simulink model "WaveBot3Dof_Control"  (R2022b)
settings: Solver=ode45  StartTime=0  StopTime=1200  FixedStep=0.01  MaxStep=0.01  RelTol=1e-3
values from neighbouring files (symbols this model uses):
  adaptSlope = [1e-4, 1e-4, 1e-3; 5e-7, 5e-7, 5e-4]    [wecSimInputFile.m]
  FBEnable = 1    [wecSimInputFile.m]
  FFEnable = 0    [wecSimInputFile.m]
  gear_ratio_h = 12.4666    [wecSimInputFile.m]
  gear_ratio_sp = diag([12.4666, 3])    [wecSimInputFile.m]
  intGain = [0, 5e-7, 1e-7; 0 5e-6 5e-8; 0 5e-5 5e-7]    [wecSimInputFile.m]
  K = 10.96    [wecSimInputFile.m]
  Kt_h = 6.1745    [wecSimInputFile.m]
  Kt_sp = 6.1745 * eye(2)    [wecSimInputFile.m]
  m = 3    [wecSimInputFile.m]
  N_max = floor(spect.f_max/spect.df)    [wecSimInputFile.m]
  N_min = ceil(spect.f_min/spect.df)    [wecSimInputFile.m]
  objCase = 1    [wecSimInputFile.m]
  OpenLoopGains = [50;100;2]    [wecSimInputFile.m]
  R_h = 0.5    [wecSimInputFile.m]
  R_sp = diag([0.5,  0.5])    [wecSimInputFile.m]
  simu = simulationClass()    [wecSimInputFile.m]
  T = 300    [wecSimInputFile.m]
  threshDF = [6000;8000;375]    [wecSimInputFile.m]
  threshPTO = [1200;1200;150]    [wecSimInputFile.m]
  Ts = dt    (= 0.01)    [wecSimInputFile.m]
  w = 2*pi*spect.f.'    [wecSimInputFile.m]
  WeightAdapt = 0    [wecSimInputFile.m]
  WeightCase = [25, 0.2,0.01; 25,0.1,0.01;25,0.2,0.1]    [wecSimInputFile.m]
  Z = [931.288383881 1656.98600833 760.743138043 168.271740533 368.778972104 366.885270862 -556.942327031 -1377.9298451 -1305.0085586 758.156793041 1688.7138346 185.859065593 ... (4023 elements, 3x3x447)]    [Z_included.mat]
  Zi_frf_AT = interp_impedance(Z,f_vec*2*pi,w)    [wecSimInputFile.m]
undefined symbols (not defined in the file or in its folder): body, constraint, Constraints, DiscIntNeverNeededParam, Floating, geometry, hydroData, mooring, spect, WECSim_Lib, WECSim_Lib_Constraints, X, Y
libraries: nesl_utility x28, sm_lib x14, simulink x6, WECSim_Lib_Frames x1, WECSim_Lib_Moorings x1, WECSim_Lib_Body_Elements x1, dspxfrm3 x1, matrix_library x1, dspsigops x1
(part 2 of 2)

== system WaveBot3Dof_Control/Subsystem/Autotuner/PTO Weight Integrator Logic/Triggered Subsystem ==
  Trigger : TriggerPort  VariantControl=Variant
  Constant : Constant  Value=0
  Constant1 : Constant
  Plus : Sum
  Out1 : Outport
  wires:
  Plus/1 -> Out1/1
  Constant/1 -> Plus/2
  Constant1/1 -> Plus/1

== system WaveBot3Dof_Control/Subsystem/Autotuner/PTO Weight Integrator Logic/Triggered Subsystem1 ==
  Trigger : TriggerPort  VariantControl=Variant
  Constant : Constant  Value=0
  Constant1 : Constant
  Plus : Sum
  Out1 : Outport
  wires:
  Plus/1 -> Out1/1
  Constant/1 -> Plus/2
  Constant1/1 -> Plus/1

== system WaveBot3Dof_Control/Subsystem/Autotuner/PTO Weight Integrator Logic/Triggered Subsystem2 ==
  Trigger : TriggerPort  VariantControl=Variant
  Constant : Constant  Value=0
  Constant1 : Constant
  Plus : Sum
  Out1 : Outport
  wires:
  Plus/1 -> Out1/1
  Constant/1 -> Plus/2
  Constant1/1 -> Plus/1

== matlab function WaveBot3Dof_Control/Subsystem/Subsystem/MATLAB Function ==
  data: vel input; Fdes output; pos input; gains input
function Fdes = PI_D_Controller(vel,pos,gains)

Fdes = zeros(3,1); % initialize output
Kp = zeros(3,1);
Ki = zeros(3,1);
D = zeros(3,1);
K = zeros(3,1); 

% build control vectors
Kp(:,1) = gains(1:2:5);
Ki(:,1) = gains(2:2:6);

% multiply elementwise by vel, pos
D = Kp .* vel;
K = Ki .* pos;

% sum according to convention
Fdes = D + K;

== matlab function WaveBot3Dof_Control/Subsystem/Autotuner/Spectral Estimation/MATLAB Function ==
  data: in1 input; Fexc output; Zi_frf_AT parameter
function Fexc = fcn(in1,  Zi_frf_AT)

F = in1(:,4:6);
V = in1(:,1:3);

Fexc = 0*F(:,[1:3]);%zeros(1,spect.N_freq);

for ii = 1:length(Fexc)
    
    % use heave only estimate 
    %Fexc(ii,1) = 2 *( Y_inv(1,:,ii)*V(ii,:).' - F(ii,1).' );%* H_inv(ii,:)
    
    % use full estimate
    Fexc(ii,:) = 2 *( Zi_frf_AT(:,:,ii)*V(ii,:).' - F(ii,:).' );
    % ETA(ii) = [1,1,1]*Y_inv(:,:,ii)*V(ii,:).';
end

% ETA = F;

== matlab function WaveBot3Dof_Control/Subsystem/Autotuner/MATLAB Function1 ==
  data: Fe input; optGains output; initGuess input; nextInit output; Kt_h parameter; R_h parameter; w parameter; Zi_frf_AT parameter; gear_ratio_h parameter; Kt_sp parameter; R_sp parameter; gear_ratio_sp parameter; m parameter; K parameter; T parameter; Weights input; PTO_h output; PTO_sp output; Df_h output; Df_sp output
function [optGains,nextInit, PTO_h, PTO_sp, Df_h, Df_sp] = gainOptimizer(Fe,initGuess,...
    Kt_h,R_h, w, Zi_frf_AT, gear_ratio_h, Kt_sp, R_sp, gear_ratio_sp, m, K, T, Weights)
% R_h = 0;
% unfortunately we must declare options every time we run
options = optimset('Display','off', 'MaxFunEvals', 1e4, 'MaxIter', 1e4);%
% further, apparently code generation cannot handle specified TolX and
% TolFun. Defaults, however, do seem adequate.

% initialize:
optGains=zeros(6,1); % initialize estimate (6 for diag only, 8 for CC)
nextInit=optGains;
cost_h = 1i; cost_sp = 1i;
exitFlag_h = 0; exitFlag_sp = 0; 
PTO_h = 0 ;
PT0_sp = zeros(2,1);
Df_h = 0; 
Df_sp = zeros(2,1);

%% break up impedance model by DOF '

% for heave only (this is not coupled to other DOFs)
Zi_frf_h=Zi_frf_AT(2,2,:);

% for surge and pitch (these are coupled)
Zi_frf_sp=Zi_frf_AT([1,3],[1,3],:);

% transpose necessary for dimensions to work out
Fe_h=Fe(:,2).';
Fe_sp=Fe(:,[1,3]).';

%% set up optimizer
cost_fun_h = @(x_h) WaveBot_power(Zi_frf_h, Fe_h, ...
    PI_FB_SISO_controller_FRF(x_h, w) , Kt_h, R_h, gear_ratio_h,Weights, m, K, T,w);

% optimize heave controller
[optGains([3,4],1)]= fminsearch(cost_fun_h, [-1000,500], options); % here a static initial guess is used: during sim ramp-up changing initial guess can be unstable

cost_fun_sp_d=@(x_sp) WaveBot_power(Zi_frf_sp, Fe_sp,...
    PI_FB_MIMO_D_controller_FRF(x_sp, w) , Kt_sp, R_sp, gear_ratio_sp,Weights, m, K, T,[w,w]);

% optimize surge/pitch controller
[optGains([1,2,5,6],1)]=fminsearch(cost_fun_sp_d, initGuess([1,2,5,6],1), options);

% output spectral info for weight adjustment
[~, ~, ~, ~, PTO_h, Df_h] = WaveBot_powerH(Zi_frf_h,Fe_h,PI_FB_SISO_controller_FRF(optGains([3,4],1), w), Kt_h, R_h, gear_ratio_h, Weights, m, K, T, w);
[~, ~, ~, ~, PTO_sp, Df_sp] = WaveBot_powerSP(Zi_frf_sp,Fe_sp, PI_FB_MIMO_D_controller_FRF(optGains([1,2,5,6],1), w), Kt_sp, R_sp, gear_ratio_sp, Weights, m, K, T, [w,w]);

% update initial guess for next time
nextInit=optGains;

% Single input single output controller for heave
    function C_h = PI_FB_SISO_controller_FRF(x_h, w)
        C_h=1i*ones(1,1,length(w)); 
        
        Kp = x_h(1);
        Ki = x_h(2);
        w = w(:);
        
        C_h(1,1,:) = Kp - 1i*Ki./w;
        
    end

% 2 input 2 output controller for surge-pitch control
    function C_sp = PI_FB_MIMO_D_controller_FRF(x_sp, w)
        C_sp=1i*ones(2,2,length(w)); C_sp(2,1)=0; C_sp(1,2)=C_sp(2,1);
        
        Kp_s = x_sp(1);
        Ki_s = x_sp(2);
        Kp_p = x_sp(3);
        Ki_p = x_sp(4);
        w = w(:);

        C_sp(1,1,:) = Kp_s - 1i*Ki_s./w;
        C_sp(2,2,:) = Kp_p - 1i*Ki_p./w;
    end
 
% optimizer runs this version
 function [Cost2, P, Cost1, Omega, Loads, Df]= WaveBot_power(Zi, Fe, C, Kt, R, gear_ratio, Weights, m, K, T, w)
        
     % initialize
        N_freq = size(Zi,3);
        P=0;
        P_f = 1i*ones(N_freq,1);
        Omega = 1i*ones(length(R),N_freq);
        Df = 0; 
        CF = 1i * ones(length(R),N_freq);
        TF = 1i * ones(length(R),N_freq);
        m0=0; 
        m2= 0; 
        v_up = 0; 
        Loads = 0; 
        Cost1 = 0; 
        Cost2 = 0; 
        
        if length(R)>1
            Weights2=Weights([1,3],:);  % if 2 DOF, pulls surge/pitch weights 
            Weights2(2,end) = -1.* Weights2(2,end);
        else
            Weights2=Weights(2,:);% if 1 DOF, pulls heave weights
        end
            Ke = Kt*2/3;
        
        for ii = 1:N_freq
            
            Omega(:,ii) = ( Zi(:,:,ii) - C(:,:,ii)) \ Fe(:,ii);
            P_f(ii) = ( (Ke*gear_ratio + (R/(gear_ratio*Kt))*C(:,:,ii)) * Omega(:,ii) )'...
                * ( ((gear_ratio*Kt)\C(:,:,ii)*Omega(:,ii)) );
            CF(:,ii)=abs(C(:,:,ii)*Omega(:,ii)); % controller force
            TF(:,ii)=(Fe(:,ii) + C(:,:,ii)*Omega(:,ii)); % total force
        end
        
        % calculate spectral moments of stress spectra
        m0 = trapz(w(:,1),abs(TF).^2,2);
        m2 = trapz(w(:,1),w.^2 .* abs((TF).^2).').';
        
        %calculate mean upcrossing time
        v_up = (1./(2*pi)).*sqrt(m2./m0);
        
        % calculate the standard deviation of the process
        sigma = sqrt(m0./length(w));
        
        % calculate the accumulated fatigue damage
        Df = (v_up.*T./K) .* (2*sqrt(2) .* sigma).^m .* gamma((m/2)+1);
        
        % calculate cost function
        P = sum(real(P_f))*3;
        Loads = sum(CF,2);
        Cost1 = real(Weights2(1,1)*P + Weights2(:,2).'*Loads);
        Cost2 = real(Weights2(1,1)*P + Weights2(:,2).'*Loads + Weights2(:,3).'*Df); 

 end

% the next two functions are basically repeats of the above, but are
% necessary to avoid size errors by the simulink code compiler

function [Cost2, P, Cost1, Omega, Loads, Df]= WaveBot_powerH(Zi, Fe, C, Kt, R, gear_ratio, Weights, m, K, T, w)
        % this includes all equally weighted loads
        % N_dof = length(R);
        % initialize all parameters/outputs
        N_freq = size(Zi,3);
        P=0;
        P_f = 1i*ones(N_freq,1);
        Omega = 1i*ones(length(R),N_freq);
        Df = 0; 
        CF = 1i * ones(length(R),N_freq);
        TF = 1i * ones(length(R),N_freq);
        sigma = 0;
        m0 = 0; 
        m2 = 0; 
        v_up = 0; 
        Loads = 0;
        Cost1 = 0; 
        Cost2 = 0;
        
        if length(R)>1
            Weights2=Weights([1,3],:); % if 2 DOF, pulls surge/pitch weights 
            Weights2(2,end) = -1.* Weights2(2,end); % to align with WS sign convention on pitch force
        else
            Weights2=Weights(2,:); % if 1 DOF, pulls heave weights
        end
            Ke = Kt*2/3;
        
        for ii = 1:N_freq
            
            Omega(:,ii) = ( Zi(:,:,ii) - C(:,:,ii)) \ Fe(:,ii);
            P_f(ii) = ( (Ke*gear_ratio + (R/(gear_ratio*Kt))*C(:,:,ii)) * Omega(:,ii) )'...
                * ( ((gear_ratio*Kt)\C(:,:,ii)*Omega(:,ii)) );
            CF(:,ii)=abs(C(:,:,ii)*Omega(:,ii)); % controller force
            TF(:,ii)=(Fe(:,ii) + C(:,:,ii)*Omega(:,ii)); % total force
        end
        
        % calculate spectral moments of stress spectra
        m0 = trapz(w(:,1),abs(TF).^2,2);
        m2 = trapz(w(:,1),w.^2 .* abs((TF).^2).').';
        
        %calculate mean upcrossing time
        v_up = (1./(2*pi)).*sqrt(m2./m0);
        
        % calculate the standard deviation of the process
        sigma = sqrt(m0./length(w));
        
        % calculate the accumulated fatigue damage
        Df = (v_up.*T./K) .* (2*sqrt(2) .* sigma).^m .* gamma((m/2)+1);
        
        if isnan(Df); % this catches the zero excitation case, which has an undefined zero-crossing time v_up
            Df = 0;
        end
        
        P = double(sum(real(P_f))*3);
        Loads = real(sum(CF,2));
        Cost1 = real(Weights2(1,1)*P + Weights2(:,2).'*Loads);
        Cost2 = real(Weights2(1,1)*P + Weights2(:,2).'*Loads + Weights2(:,3).'*Df); % additional penalty for reactive terms.
    end

function [Cost2, P, Cost1, Omega, Loads, Df]= WaveBot_powerSP(Zi, Fe, C, Kt, R, gear_ratio, Weights, m, K, T, w)

        N_freq = size(Zi,3);
        P=0;
        P_f = 1i*ones(N_freq,1);
        Omega = 1i*ones(length(R),N_freq);
        Df = zeros(2,1); 
        CF = 1i * ones(length(R),N_freq);
        TF = 1i * ones(length(R),N_freq);
        sigma = zeros(2,1);
        m0 = zeros(2,1); 
        m2 = zeros(2,1); 
        v_up = zeros(2,1); 
        Loads = zeros(2,1);
        Cost1 = zeros(2,1); 
        Cost2 = zeros(2,1);
        
        if length(R)>1
            Weights2=Weights([1,3],:);
            Weights2(2,end) = -1.* Weights2(2,end);
        else
            Weights2=Weights(2,:);
        end
            Ke = Kt*2/3;
        
        for ii = 1:N_freq
            
            Omega(:,ii) = ( Zi(:,:,ii) - C(:,:,ii)) \ Fe(:,ii);
            P_f(ii) = ( (Ke*gear_ratio + (R/(gear_ratio*Kt))*C(:,:,ii)) * Omega(:,ii) )'...
                * ( ((gear_ratio*Kt)\C(:,:,ii)*Omega(:,ii)) );
            CF(:,ii)=abs(C(:,:,ii)*Omega(:,ii)); % controller force
            TF(:,ii)=(Fe(:,ii) + C(:,:,ii)*Omega(:,ii)); % total force
        end
        
        % calculate spectral moments of stress spectra
        m0 = trapz(w(:,1),abs(TF).^2,2);
        m2 = trapz(w(:,1),w.^2 .* abs((TF).^2).').';
        
        %calculate mean upcrossing time
        v_up = (1./(2*pi)).*sqrt(m2./m0);
        
        % calculate the standard deviation of the process
        sigma = sqrt(m0./length(w));
        
        % calculate the accumulated fatigue damage
        Df = double((v_up.*T./K) .* (2*sqrt(2) .* sigma).^m .* gamma((m/2)+1)); 
        if any(isnan(Df))
            Df = [0;0]
        end
        
        P = sum(real(P_f))*3;
        Loads = real(sum(CF,2));
        Cost1 = real(Weights2(1,1)*P + Weights2(:,2).'*Loads);
        Cost2 = real(Weights2(1,1)*P + Weights2(:,2).'*Loads + Weights2(:,3).'*Df); 
    end


end

== matlab function WaveBot3Dof_Control/Subsystem/Autotuner/MATLAB Function2 ==
  data: F_tot input; F_des input; objCase parameter; threshPTO input; Weights output; err output; threshDF input; w parameter; adaptSlope parameter; activePTO output; activeDf output
function [Weights,err,activePTO,activeDf]  = weightTransition(F_tot, F_des, objCase, threshPTO, threshDF, w, adaptSlope)

% F_des : the desired PTO force
% F_exc : the excitation force spectra
% objCase: Single value of set {1,2,3,4]. 1 maximize power, 2 max power and
% limit PTO load, 3 max power and limit fatigue damage, 4 max power and
% limit both PTO load and fatigue damage.
% threshPTO: the spectral power at which the PTO load minimization
% objective becomes non-zero, 3 x 1 vector for each DOF. 
% threshDF: the spectral power of total load at which the fatigue damage
% minimization objective weight becomes non-zero 3 x 1 vector for each DOF.
% w: the radian frequency vector at which V_enc, F_des, and F_tot are defined 

% initialize output and variables
Weights = zeros(3,3); % one weight per DOF * objective
%F_des = zeros(3,1);
%F_tot = zeros(3,1);
activePTO = logical(zeros(3,1)); 
activeDf = logical(zeros(3,1)); 
err = zeros(3,3);

% integrate the frequency vectors
switch objCase;
    case 1
        Weights = [25,0,0; 25,0,0; 25,0,0]; % all we care about is power
    case 2
        Weights = [25,0,0; 25,0,0; 25,0,0]; % all we care about is power unless threshold exceeded
        activePTO = F_des > threshPTO;
        % tuned from opt power gains at 2,10
        err(1,2) = real(F_des(1)) - threshPTO(1);
        err(2,2) = real(F_des(2)) - threshPTO(2);
        err(3,2) = real(F_des(3)) - threshPTO(3);
        Weights(1,2) = adaptSlope(1,1) * activePTO(1) * (real(F_des(1)) - threshPTO(1));
        Weights(2,2) = adaptSlope(1,2) * activePTO(2) * (real(F_des(2)) - threshPTO(2));
        Weights(3,2) = adaptSlope(1,3) * activePTO(3) * (real(F_des(3)) - threshPTO(3));
               
    case 3
        Weights = [25,0,0; 25,0,0; 25,0,0]; % all we care about is power unless threshold exceeded
        activeDf = F_tot > threshDF;
        err(1,3) = real(F_tot(1)) - threshDF(1);
        err(2,3) = real(F_tot(2)) - threshDF(2);
        err(3,3) = real(F_tot(3)) - threshDF(3);
        Weights(1,3) = adaptSlope(2,1)* activeDf(1) * (real(F_tot(1)) - threshDF(1));
        Weights(2,3) = adaptSlope(2,2) * activeDf(2) * (real(F_tot(2)) - threshDF(2));
        Weights(3,3) = adaptSlope(2,3) * activeDf(3) * (real(F_tot(3)) - threshDF(3));
        
    case 4
         Weights = [25,0,0; 25,0,0; 25,0,0]; % all we care about is power unless threshold exceeded
        activePTO = F_des > threshPTO;
        activeDf = F_tot > threshDF;
        err(1,2) = real(F_des(1)) - threshPTO(1);
        err(2,2) = real(F_des(2)) - threshPTO(2);
        err(3,2) = real(F_des(3)) - threshPTO(3);
        err(1,3) = real(F_tot(1)) - threshDF(1);
        err(2,3) = real(F_tot(2)) - threshDF(2);
        err(3,3) = real(F_tot(3)) - threshDF(3);
        Weights(1,2) = adaptSlope(1,1) * activePTO(1) * (real(F_des(1)) - threshPTO(1));
        Weights(2,2) = adaptSlope(1,2) * activePTO(2) * (real(F_des(2)) - threshPTO(2));
        Weights(3,2) = adaptSlope(1,3) * activePTO(3) * (real(F_des(3)) - threshPTO(3));
        Weights(1,3) = adaptSlope(2,1) * activeDf(1) * (real(F_tot(1)) - threshDF(1));
        Weights(2,3) = adaptSlope(2,2) * activeDf(2) * (real(F_tot(2)) - threshDF(2));
        Weights(3,3) = adaptSlope(2,3) * activeDf(3) * (real(F_tot(3)) - threshDF(3));

end
